simulink model "kalmanfilter"  (R2023b)
settings: Solver=VariableStepAuto  StartTime=0.0  StopTime=10.0  RelTol=1e-3
settings Model: Creator=54238  LastModifiedBy=54238
settings RTWCC: GPUComputeCapability=5.0

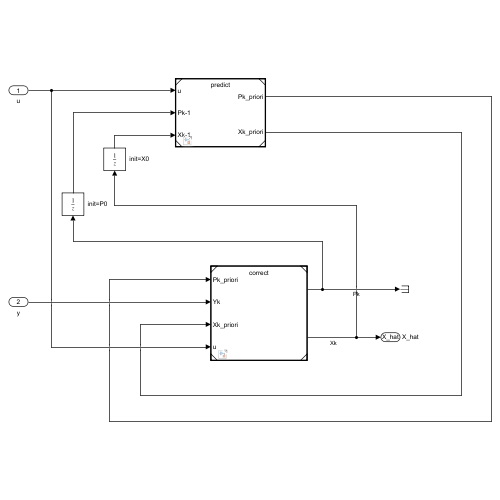
[thumbnail: Simulink's stored preview of the top-level diagram]
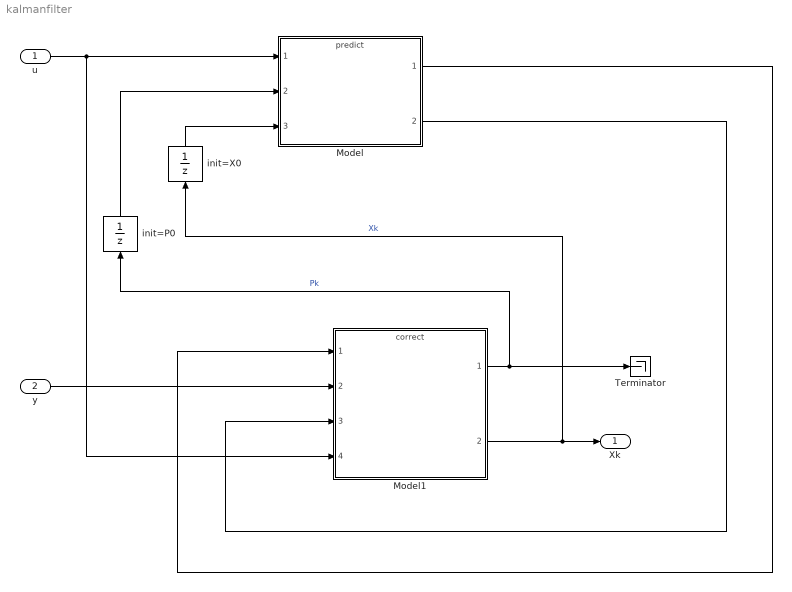
== system kalmanfilter ==
  u : Inport
  y : Inport  Port=2
  Model : ModelReference  ModelNameDialog=predict.slx  SimulationMode=Normal  ModelReferenceVersion=1.4
  Model1 : ModelReference  ModelNameDialog=correct.slx  SimulationMode=Normal  ModelReferenceVersion=1.4
  Terminator : Terminator
  init=P0 : UnitDelay  SampleTime=-1  StateName=p0  HasFrameUpgradeWarning=on
  init=X0 : UnitDelay  SampleTime=-1  HasFrameUpgradeWarning=on
  Xk : Outport  SignalName=X_hat
  wires:
  u/1 -> Model1/4, Model/1
  init=P0/1 -> Model/2
  init=X0/1 -> Model/3
  y/1 -> Model1/2
  Model1/1 -> init=P0/1, Terminator/1  "Pk"
  Model1/2 -> Xk/1, init=X0/1  "Xk"
  Model/1 -> Model1/1
  Model/2 -> Model1/3
